simulink model "lv_fcnCp"  (Simulink 7.1)
settings: Solver=ode45  StartTime=0.0  StopTime=100  RelTol=1e-3
settings Model: Creator=lv  LastModifiedBy=lv

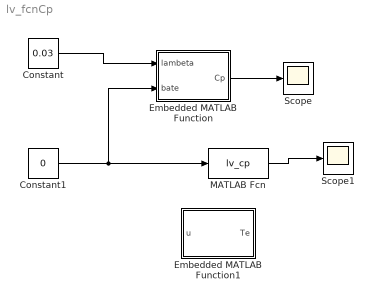
== system lv_fcnCp ==
  Constant : Constant  Value=0.03  OutDataType=sfix(16)  OutScaling=2^0
  Constant1 : Constant  Value=0  OutDataType=sfix(16)  OutScaling=2^0
  Embedded MATLAB Function : Stateflow chart
  Embedded MATLAB Function1 : Stateflow chart
  MATLAB Fcn : MATLABFcn  MATLABFcn=lv_cp
  Scope : Scope
  Scope1 : Scope
  wires:
  Constant/1 -> Embedded MATLAB Function/1(lambeta)
  Embedded MATLAB Function/1(Cp) -> Scope/1
  Constant1/1 -> MATLAB Fcn/1, Embedded MATLAB Function/2(bate)
  MATLAB Fcn/1 -> Scope1/1

== matlab function Embedded MATLAB Function1 ==
  data: u input double; Te output double
function Te= fcn(u)
% This block supports the Embedded MATLAB subset.
% See the help menu for details. 

Te = 1*u;

== matlab function Embedded MATLAB Function ==
  data: lambeta input double; Cp output double; bate input double
function Cp = fcn(lambeta,bate)
%#eml
% a=0;
% b=0;
% Cp=pi;
% Cp=(0.44-0.0167*b)*sin(pi*(a-3)/(15-0.3*b))-0.00184*(a-3)*b;
Cp=(0.44-0.0167*bate)*sin(pi*(lambeta-3)/(15-0.3*bate))-0.00184*(lambeta-3)*bate;
% Cp=lambeta+bate;
